simulink model "LaoWang_chap8_lqr"  (R2022a)
settings: Solver=VariableStepAuto  StartTime=0.0  StopTime=100  RelTol=1e-3
libraries: Solver_SF x1
settings Model: Creator=HaiChen  LastModifiedBy=HaiChen

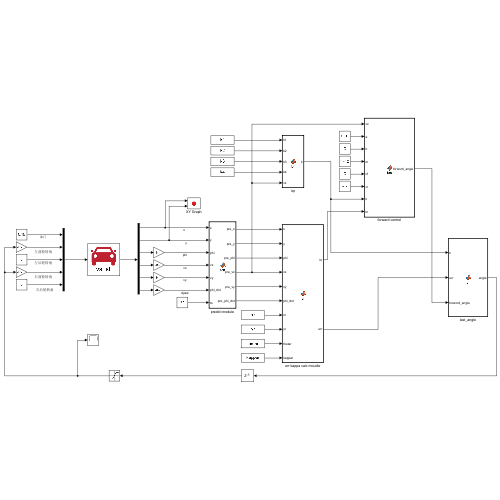
[thumbnail: Simulink's stored preview of the top-level diagram]
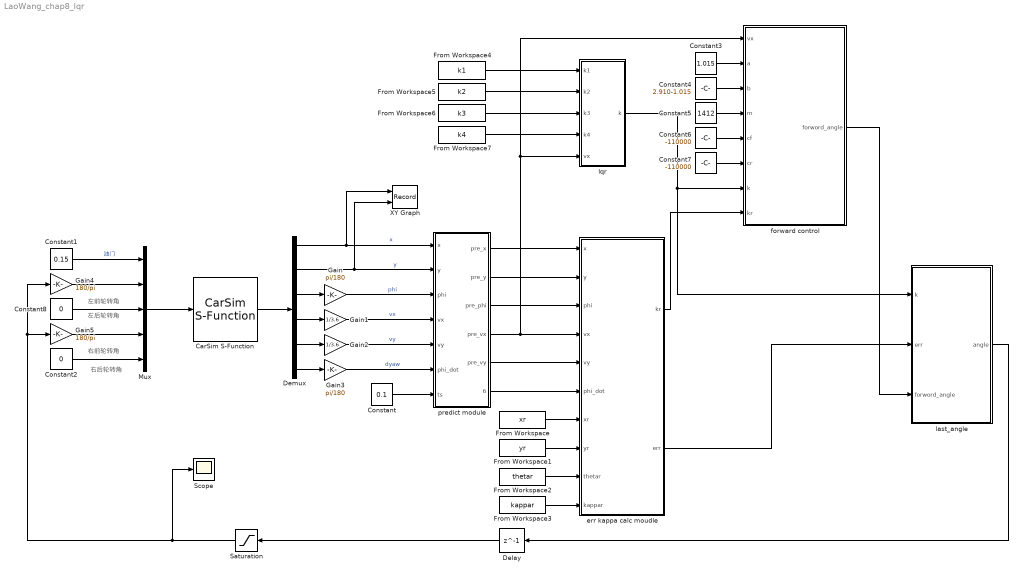
== system LaoWang_chap8_lqr ==
  note: 左后轮转角
  note: 左前轮转角
  note: 右前轮转角
  note: 右后轮转角
  CarSim S-Function : Solver_SF/CarSim S-Function  Priority=1  SIMFILE=LaoWang_chap8_lqr.sim
  Constant : Constant  Value=0.1
  Constant1 : Constant  Value=0.15
  Constant2 : Constant  Value=0
  Constant3 : Constant  Value=1.015
  Constant4 : Constant  Value=2.910-1.015
  Constant5 : Constant  Value=1412
  Constant6 : Constant  Value=-110000
  Constant7 : Constant  Value=-110000
  Constant8 : Constant  Value=0
  Delay : Delay  DelayLength=1
  Demux : Demux  Outputs=6
  From Workspace : FromWorkspace  VariableName=xr
  From Workspace1 : FromWorkspace  VariableName=yr
  From Workspace2 : FromWorkspace  VariableName=thetar
  From Workspace3 : FromWorkspace  VariableName=kappar
  From Workspace4 : FromWorkspace  VariableName=k1
  From Workspace5 : FromWorkspace  VariableName=k2
  From Workspace6 : FromWorkspace  VariableName=k3
  From Workspace7 : FromWorkspace  VariableName=k4
  Gain : Gain  Gain=pi/180
  Gain1 : Gain  Gain=1/3.6
  Gain2 : Gain  Gain=1/3.6
  Gain3 : Gain  Gain=pi/180
  Gain4 : Gain  Gain=180/pi
  Gain5 : Gain  Gain=180/pi
  Mux : Mux  Inputs=5
  Saturation : Saturate  UpperLimit=1  LowerLimit=-1
  Scope : Scope
  XY Graph : Record  FileSettingsInternal="{\"entries\":[{\"content\":{\"excelSettings\":{\"content\":{},\"type\":\"Streamout.ExcelSettings\"}},\"type\":\"Streamout.FileSettingStorage\",\"uuid\":\"333ade27-daaf-48fc-95cc-648013fd297e\"}],\"packageUris\":[\"http://schema.mathworks.com/mf0/streamout_blocks/R2020a\"],\"version\":\"1.0\"}"  Layout=[1 1]  SignalsInternal="{\"entries\":[{\"content\":{\"signals\":[{\"content\":{\"blockPath\":[\"LaoWang_chap8_lqr/XY Graph\"],\"channel\":[],\"dimensions\":[1],\"domain\":\"LaoWang_chap8_lqr/XY Graph\",\"lineColor\":\"#a2142f\",\"plots\":[1],\"port\":1,\"sid\":[\"\"],\"signalID\":605,\"signalName\":\"x\"},\"type\":\"RecordBlkView.Signal\",\"uuid\":\"d6d6934b-4596-4759-a39d-c71adecb1ea4\"},{\"content\":{\"blockPath\":[\"LaoWang_chap8_lqr/XY Graph\"],\"channel\":[],\"dimensions\":[1],\"domain\":\"LaoWang_chap8_lqr/XY Graph\",\"lineColor\":\"#139fff\",\"plots\":[1],\"port\":2,\"sid\":[\"\"],\"signalID\":609,\"signalName\":\"y\"},\"type\":\"RecordBlkView.Signal\",\"uuid\":\"0e2dbc68-aa6a-4af3-85d4-265a3f7afe98\"}]},\"type\":\"RecordBlkView.InputSignals\",\"uuid\":\"a4d6e0d1-ed74-47d6-9560-4e6e709edafd\"}],\"packageUris\":[\"http://schema.mathworks.com/mf0/streamout_blocks/R2020a\"],\"version\":\"1.0\"}"  VisualizationBindings="{\"xyplotplugin\":{\"info\":[{\"series\":[{\"bindingParametersList\":[{\"parameter\":\"X-Axis\",\"signalID\":605,\"signalName\":\"x\"},{\"parameter\":\"Y-Axis\",\"signalID\":609,\"signalName\":\"y\"}],\"seriesID\":32386}],\"subplotID\":1}]}}"  CompatibilityTag=XY
  err kappa calc moudle : MATLAB Function  TreatAsAtomicUnit=on
  forward control : MATLAB Function  TreatAsAtomicUnit=on
  last_angle : MATLAB Function  TreatAsAtomicUnit=on
  lqr : MATLAB Function  TreatAsAtomicUnit=on
  predict module : MATLAB Function  TreatAsAtomicUnit=on
  wires:
  Mux/1 -> CarSim S-Function/1
  Demux/3 -> Gain/1
  Demux/4 -> Gain1/1
  Demux/2 -> XY Graph/2, predict module/2(y)  "y"
  Demux/1 -> XY Graph/1, predict module/1(x)  "x"
  CarSim S-Function/1 -> Demux/1
  Demux/5 -> Gain2/1
  Demux/6 -> Gain3/1
  Gain/1 -> predict module/3(phi)  "phi"
  Gain1/1 -> predict module/4(vx)  "vx"
  Gain2/1 -> predict module/5(vy)  "vy"
  Gain3/1 -> predict module/6(phi_dot)  "dyaw"
  Constant/1 -> predict module/7(ts)
  predict module/1(pre_x) -> err kappa calc moudle/1(x)
  predict module/2(pre_y) -> err kappa calc moudle/2(y)
  predict module/3(pre_phi) -> err kappa calc moudle/3(phi)
  predict module/4(pre_vx) -> err kappa calc moudle/4(vx), forward control/1(vx), lqr/5(vx)
  predict module/5(pre_vy) -> err kappa calc moudle/5(vy)
  predict module/6(pre_phi_dot) -> err kappa calc moudle/6(phi_dot)
  From Workspace/1 -> err kappa calc moudle/7(xr)
  From Workspace1/1 -> err kappa calc moudle/8(yr)
  From Workspace2/1 -> err kappa calc moudle/9(thetar)
  From Workspace3/1 -> err kappa calc moudle/10(kappar)
  From Workspace4/1 -> lqr/1(k1)
  From Workspace5/1 -> lqr/2(k2)
  From Workspace6/1 -> lqr/3(k3)
  From Workspace7/1 -> lqr/4(k4)
  lqr/1(k) -> last_angle/1(k), forward control/7(k)
  err kappa calc moudle/1(kr) -> forward control/8(kr)
  forward control/1(forword_angle) -> last_angle/3(forword_angle)
  err kappa calc moudle/2(err) -> last_angle/2(err)
  last_angle/1(angle) -> Delay/1
  Constant1/1 -> Mux/1  "油门"
  Delay/1 -> Saturation/1
  Constant2/1 -> Mux/5
  Constant3/1 -> forward control/2(a)
  Constant4/1 -> forward control/3(b)
  Constant5/1 -> forward control/4(m)
  Constant6/1 -> forward control/5(cf)
  Constant7/1 -> forward control/6(cr)
  Gain4/1 -> Mux/2
  Saturation/1 -> Scope/1, Gain4/1, Gain5/1
  Gain5/1 -> Mux/4
  Constant8/1 -> Mux/3

== matlab function LaoWang_chap8_lqr/err kappa calc moudle ==
  data: x input; kr output; y input; phi input; vx input; vy input; phi_dot input; xr input; yr input; thetar input; kappar input; err output
function [kr,err] = fcn(x,y,phi,vx,vy,phi_dot,xr,yr,thetar,kappar)
    n=length(xr);%先找到规划轨迹的长度，共有多少个规划点
    d_min=(x-xr(1))^2+(y-yr(1))^2;%把最短距离设为真实位置与第1个点。可以不用开平方根，减少计算量，因为并不关心距离是多少，只想找到最短点的序号
    min=1;%先把最短点的序号设为1
    for i=1:n%遍历所有的点
        d=(x-xr(i))^2+(y-yr(i))^2;%计算它与真实的位置的之间的距离
        if d<d_min%如果能找到比所设置的最短距离还要短
            d_min=d;%将值赋为最短距离
            min=i;%把序点的序号赋给min
        end
    end
    %遍历一遍后，一定能找到最短的距离规划点的序号，其实就是选择排序法
    dmin=min;
    tor=[cos(thetar(dmin));sin(thetar(dmin))];
    nor=[-sin(thetar(dmin));cos(thetar(dmin))];
    d_err=[x-xr(dmin);y-yr(dmin)];
    ed=nor'*d_err;
    es=tor'*d_err;
%     projection_point_thetar=thetar(dmin);%apollo
    projection_point_thetar=thetar(dmin)+kappar(dmin)*es;%投影点的航向角
    ed_dot=vy*cos(phi-projection_point_thetar)+vx*sin(phi-projection_point_thetar);
    %%%%%%%%%
    ephi=sin(phi-projection_point_thetar);%因为角度具有多值性，使用sin来消除因为多2pi或者少2pi而导致的算法出错
    %%%%%%%%%
    s_dot=vx*cos(phi-projection_point_thetar)-vy*sin(phi-projection_point_thetar);
    s_dot=s_dot/(1-kappar(dmin)*ed);
    ephi_dot=phi_dot-kappar(dmin)*s_dot;
    kr=kappar(dmin);
    err=[ed;ed_dot;ephi;ephi_dot];
end

== matlab function LaoWang_chap8_lqr/predict module ==
  data: x input; pre_x output; y input; phi input; vx input; vy input; phi_dot input; ts input; pre_y output; pre_phi output; pre_vx output; pre_vy output; pre_phi_dot output
function [ pre_x,pre_y,pre_phi,pre_vx,pre_vy,pre_phi_dot] = fcn(x,y,phi,vx,vy,phi_dot,ts)
    pre_x = x + vx*ts*cos(phi) - vy*ts*sin(phi);
    pre_y = y + vy*ts*cos(phi) + vx*ts*sin(phi);
    pre_phi = phi + phi_dot*ts;
    pre_vx = vx;
    pre_vy = vy;
    pre_phi_dot = phi_dot;
end

== matlab function LaoWang_chap8_lqr/lqr ==
  data: k1 input; k output; k2 input; k3 input; k4 input; vx input
function k  = fcn(k1,k2,k3,k4,vx)
    if abs(vx)<0.01%特殊处理如果 v 的绝对值小于0.01，
        k=[0,0,0,0];%直接令 k 就等于0，它是航向量
    else
        index=round(vx/0.01);%否则的话就用 v x 除001，再用round四舍五入，值就是所要的匹配的序号
        k=[k1(index),k2(index),k3(index),k4(index)];
    end
end

== matlab function LaoWang_chap8_lqr/forward control ==
  data: vx input; forword_angle output; a input; b input; m input; cf input; cr input; k input; kr input
function forword_angle = fcn(vx,a,b,m,cf,cr,k,kr)
    forword_angle=kr*(a+b-b*k(3)-(m*vx*vx/(a+b))*((b/cf)+(a/cr)*k(3)-(a/cr)));
end

== matlab function LaoWang_chap8_lqr/last_angle ==
  data: k input; angle output; err input; forword_angle input
function angle = fcn(k,err,forword_angle)
    angle=-k*err+forword_angle;
end
